simulink model "TorqueControl_QuadRad_MPC_03_FMINCON"  (R2015b)
settings: Solver=FixedStepAuto  StartTime=0.0  StopTime=100  FixedStep=1  RelTol=1e-3
values from neighbouring files (symbols this model uses):
  bicycle = initBicycle(60, 0.01468, 0.79, 0.33, 0.17, 5.5, 24, 50, 48)    [RunSimulinkSim_MPC.m]
  cyclist = initCyclist(0, 30, 183, 75, 80)    [RunSimulinkSim_MPC.m]
  environment = initEnvironment_V2(altitude, distance, fRES, 9.81, 1.2041)    [RunSimulinkSim_MPC.m]
  system = initHRmodel(0.0113, 0.0072, 0.0049, 0.0041, 19.8002, 0.0072, cyclist.P_max, cyclist.cadence)    [RunSimulinkSim_MPC.m]
undefined symbols (not defined in the file or in its folder): init
libraries: simulink x2, aerolibconvert2 x1
settings Model: Creator=Daniel  LastModifiedBy=Daniel
settings DataIOCC: SaveFormat=Array

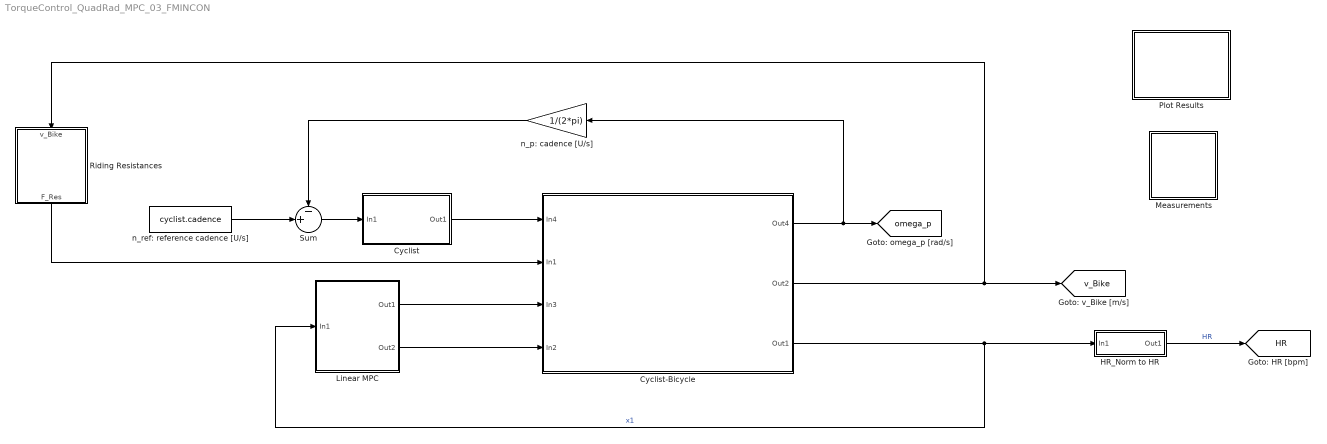
== system TorqueControl_QuadRad_MPC_03_FMINCON ==
  Cyclist : Subsystem
  Cyclist-Bicycle : Subsystem
  HR_Norm to HR : Subsystem
  Linear MPC : Subsystem
  Measurements : Subsystem
  Plot Results : Subsystem
  Riding Resistances : Subsystem
  Sum : Sum  Inputs=-+|
  n_p: cadence [U/s] : Gain  Gain=1/(2*pi)
  n_ref: reference cadence [U/s] : Constant  Value=cyclist.cadence
  tag scope: HR=global, omega_p=global, v_Bike=global
  wires:
  Linear MPC/1(Out1) -> Cyclist-Bicycle/3(In3)
  Cyclist-Bicycle/1(Out4) -> n_p: cadence [U/s]/1, [omega_p]
  n_ref: reference cadence [U/s]/1 -> Sum/2
  n_p: cadence [U/s]/1 -> Sum/1
  Riding Resistances/1(F_Res) -> Cyclist-Bicycle/2(In1)
  Cyclist-Bicycle/2(Out2) -> [v_Bike], Riding Resistances/1(v_Bike)
  Cyclist-Bicycle/3(Out1) -> Linear MPC/1(In1), HR_Norm to HR/1(In1)  "x1"
  HR_Norm to HR/1(Out1) -> [HR]  "HR"
  Sum/1 -> Cyclist/1(In1)
  Cyclist/1(Out1) -> Cyclist-Bicycle/1(In4)
  Linear MPC/2(Out2) -> Cyclist-Bicycle/4(In2)

== system TorqueControl_QuadRad_MPC_03_FMINCON/Cyclist ==
  In1 : Inport
  T_R,p: Rider torque at pedals [Nm] : simulink/Continuous/PID Controller  Controller=PID  TimeDomain=Continuous-time  SampleTime=-1  IntegratorMethod=Forward Euler  FilterMethod=Forward Euler  Form=Parallel  UseFilter=on  ControllerParametersSource=internal  P=200  I=2  D=0  N=1  InitialConditionSource=internal  InitialConditionForIntegrator=0  InitialConditionForFilter=0  ExternalReset=none  LimitOutput=on  UpperSaturationLimit=cyclist.P_max/(2*pi*2/3)  LowerSaturationLimit=0  LinearizeAsGain=on  AntiWindupMode=none  Kb=1  TrackingMode=off  Kt=1  PParamMin=[]  PParamMax=[]  IParamMin=[]  IParamMax=[]  DParamMin=[]  DParamMax=[]  NParamMin=[]  NParamMax=[]  KbParamMin=[]  KbParamMax=[]  KtParamMin=[]  KtParamMax=[]  POutMin=[]  POutMax=[]  IOutMin=[]  IOutMax=[]  DOutMin=[]  DOutMax=[]  NOutMin=[]  NOutMax=[]  KbOutMin=[]  KbOutMax=[]  KtOutMin=[]  KtOutMax=[]  IntegratorOutMin=[]  IntegratorOutMax=[]  FilterOutMin=[]  FilterOutMax=[]  SumOutMin=[]  SumOutMax=[]  SumI1OutMin=[]  SumI1OutMax=[]  SumI2OutMin=[]  SumI2OutMax=[]  SumI3OutMin=[]  SumI3OutMax=[]  SumDOutMin=[]  SumDOutMax=[]  SaturationOutMin=[]  SaturationOutMax=[]  IntegratorContinuousStateAttributes=''  IntegratorStateMustResolveToSignalObject=off  IntegratorRTWStateStorageClass=Auto  FilterContinuousStateAttributes=''  FilterStateMustResolveToSignalObject=off  FilterRTWStateStorageClass=Auto  DifferentiatorICPrevScaledInput=0  DifferentiatorOutMin=[]  DifferentiatorOutMax=[]
  Out1 : Outport
  tag scope: T_Rp=global
  wires:
  In1/1 -> T_R,p: Rider torque at pedals [Nm]/1  "e_n"
  T_R,p: Rider torque at pedals [Nm]/1 -> [T_Rp], Out1/1  "T_R,p [Nm]"

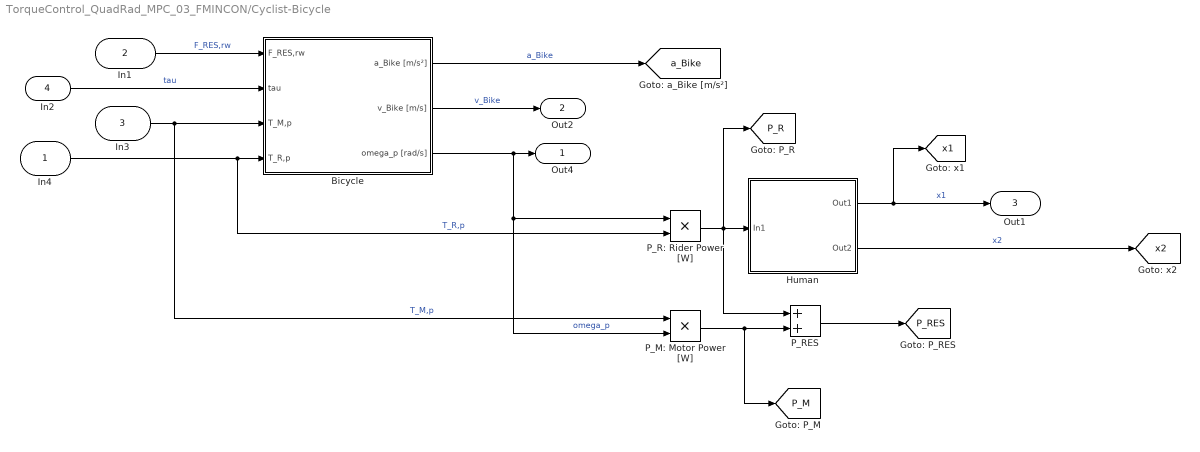
== system TorqueControl_QuadRad_MPC_03_FMINCON/Cyclist-Bicycle ==
  In4 : Inport
  In1 : Inport  Port=2
  In3 : Inport  Port=3
  In2 : Inport  Port=4
  Bicycle : Subsystem
  Human : Subsystem
  P_M: Motor Power [W] : Product
  P_R: Rider Power [W] : Product
  P_RES : Sum
  Out4 : Outport
  Out2 : Outport  Port=2
  Out1 : Outport  Port=3
  tag scope: P_M=global, P_R=global, P_RES=global, a_Bike=global, x1=global, x2=global
  wires:
  P_R: Rider Power [W]/1 -> [P_R], P_RES/1, Human/1(In1)
  Bicycle/2(v_Bike [m/s]) -> Out2/1  "v_Bike"
  Bicycle/1(a_Bike [m/s²]) -> [a_Bike]  "a_Bike"
  Human/2(Out2) -> [x2]  "x2"
  In2/1 -> Bicycle/2(tau)  "tau"
  In3/1 -> P_M: Motor Power [W]/1, Bicycle/3(T_M,p)  "T_M,p"
  In4/1 -> P_R: Rider Power [W]/2, Bicycle/4(T_R,p)  "T_R,p"
  In1/1 -> Bicycle/1(F_RES,rw)  "F_RES,rw"
  Bicycle/3(omega_p [rad/s]) -> Out4/1, P_M: Motor Power [W]/2, P_R: Rider Power [W]/1  "omega_p"
  Human/1(Out1) -> Out1/1, [x1]  "x1"
  P_M: Motor Power [W]/1 -> [P_M], P_RES/2
  P_RES/1 -> [P_RES]

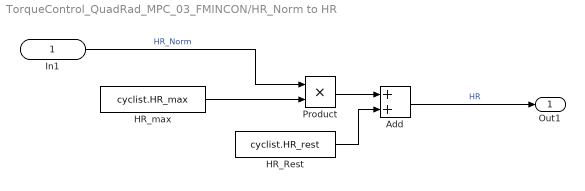
== system TorqueControl_QuadRad_MPC_03_FMINCON/HR_Norm to HR ==
  In1 : Inport
  Add : Sum
  HR_Rest : Constant  Value=cyclist.HR_rest
  HR_max : Constant  Value=cyclist.HR_max
  Product : Product
  Out1 : Outport
  wires:
  HR_max/1 -> Product/2
  Add/1 -> Out1/1  "HR"
  Product/1 -> Add/1
  HR_Rest/1 -> Add/2
  In1/1 -> Product/1  "HR_Norm"

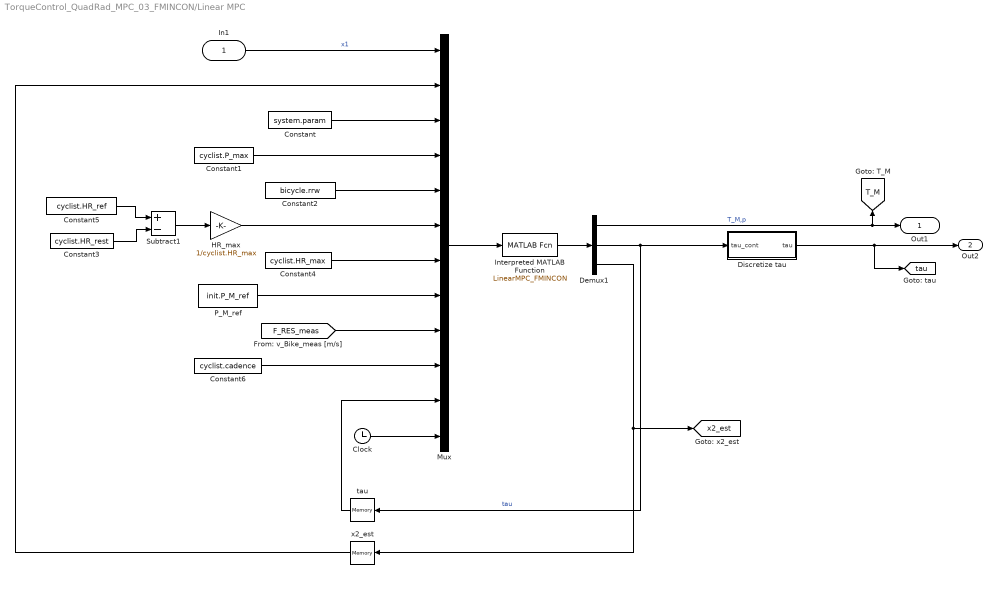
== system TorqueControl_QuadRad_MPC_03_FMINCON/Linear MPC ==
  In1 : Inport
  Clock : Clock
  Constant : Constant  Value=system.param
  Constant1 : Constant  Value=cyclist.P_max
  Constant2 : Constant  Value=bicycle.rrw
  Constant3 : Constant  Value=cyclist.HR_rest
  Constant4 : Constant  Value=cyclist.HR_max
  Constant5 : Constant  Value=cyclist.HR_ref
  Constant6 : Constant  Value=cyclist.cadence
  Demux1 : Demux  Outputs=3
  Discretize tau : MATLAB Function  TreatAsAtomicUnit=on
  HR_max : Gain  Gain=1/cyclist.HR_max
  Interpreted MATLAB Function : MATLABFcn  MATLABFcn=LinearMPC_FMINCON  OutputDimensions=3
  Mux : Mux  Inputs=12
  P_M_ref : Constant  Value=init.P_M_ref
  Subtract1 : Sum  Inputs=+-
  tau : Memory  X0=init.tau  InheritSampleTime=on
  x2_est : Memory  X0=init.x2_est  InheritSampleTime=on
  Out1 : Outport
  Out2 : Outport  Port=2
  tag scope: T_M=global, tau=global, x2_est=global
  wires:
  In1/1 -> Mux/1  "x1"
  Constant/1 -> Mux/3
  Constant1/1 -> Mux/4
  Constant2/1 -> Mux/5
  Constant5/1 -> Subtract1/1
  Constant3/1 -> Subtract1/2
  Mux/1 -> Interpreted MATLAB Function/1
  Interpreted MATLAB Function/1 -> Demux1/1
  Demux1/3 -> x2_est/1, [x2_est]
  x2_est/1 -> Mux/2
  P_M_ref/1 -> Mux/8
  [F_RES_meas] -> Mux/9
  Constant6/1 -> Mux/10
  Subtract1/1 -> HR_max/1
  HR_max/1 -> Mux/6
  Demux1/1 -> Out1/1, [T_M]  "T_M,p"
  Demux1/2 -> tau/1, Discretize tau/1(tau_cont)  "tau"
  tau/1 -> Mux/11
  Constant4/1 -> Mux/7
  Clock/1 -> Mux/12
  Discretize tau/1(tau) -> Out2/1, [tau]

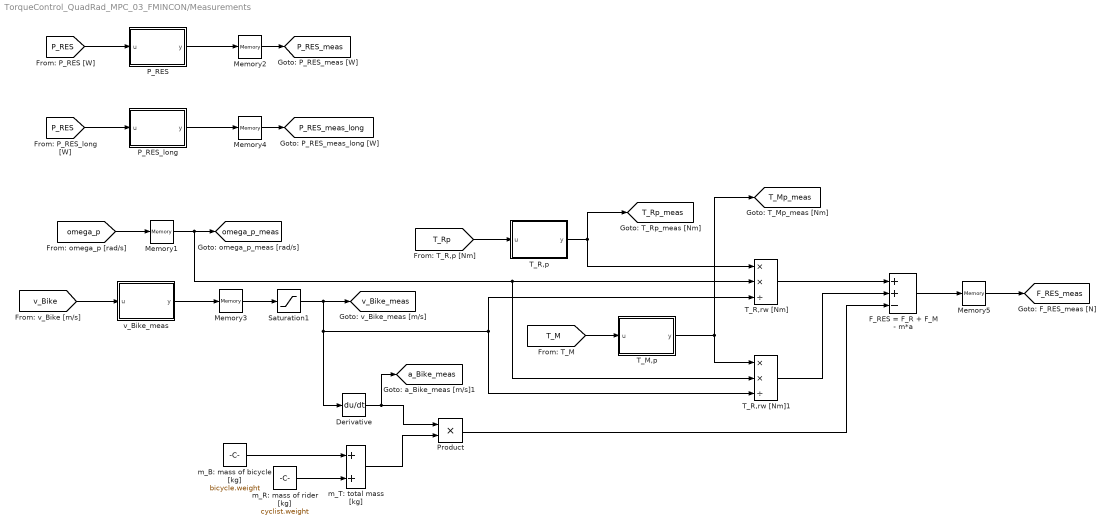
== system TorqueControl_QuadRad_MPC_03_FMINCON/Measurements ==
  Derivative : Derivative
  F_RES = F_R + F_M - m*a : Sum  Inputs=++-
  Memory1 : Memory  X0=init.omega_p  InheritSampleTime=on
  Memory2 : Memory  X0=init.P_RES  InheritSampleTime=on
  Memory3 : Memory  X0=init.v_Bike  InheritSampleTime=on
  Memory4 : Memory  X0=init.P_RES  InheritSampleTime=on
  Memory5 : Memory  X0=10  InheritSampleTime=on
  P_RES : MATLAB Function  TreatAsAtomicUnit=on
  P_RES_long : MATLAB Function  TreatAsAtomicUnit=on
  Product : Product
  Saturation1 : Saturate  UpperLimit=100  LowerLimit=0.1
  T_M,p : MATLAB Function  TreatAsAtomicUnit=on
  T_R,p : MATLAB Function  TreatAsAtomicUnit=on
  T_R,rw [Nm] : Product  Inputs=**/
  T_R,rw [Nm]1 : Product  Inputs=**/
  m_B: mass of bicycle [kg] : Constant  Value=bicycle.weight
  m_R: mass of rider [kg] : Constant  Value=cyclist.weight
  m_T: total mass [kg] : Sum
  v_Bike_meas : MATLAB Function  TreatAsAtomicUnit=on
  tag scope: F_RES_meas=global, P_RES_meas=global, P_RES_meas_long=global, T_Mp_meas=global, T_Rp_meas=global, a_Bike_meas=global, omega_p_meas=global, v_Bike_meas=global
  wires:
  [P_RES] -> P_RES/1(u)
  Memory2/1 -> [P_RES_meas]
  [omega_p] -> Memory1/1
  Memory1/1 -> T_R,rw [Nm]1/2, T_R,rw [Nm]/2, [omega_p_meas]
  P_RES/1(y) -> Memory2/1
  Memory3/1 -> Saturation1/1
  [v_Bike] -> v_Bike_meas/1(u)
  Saturation1/1 -> T_R,rw [Nm]1/3, T_R,rw [Nm]/3, Derivative/1, [v_Bike_meas]
  v_Bike_meas/1(y) -> Memory3/1
  [P_RES] -> P_RES_long/1(u)
  Memory4/1 -> [P_RES_meas_long]
  P_RES_long/1(y) -> Memory4/1
  m_B: mass of bicycle [kg]/1 -> m_T: total mass [kg]/1
  m_T: total mass [kg]/1 -> Product/2
  m_R: mass of rider [kg]/1 -> m_T: total mass [kg]/2
  Derivative/1 -> [a_Bike_meas], Product/1
  [T_Rp] -> T_R,p/1(u)
  [T_M] -> T_M,p/1(u)
  T_R,rw [Nm]/1 -> F_RES = F_R + F_M - m*a/1
  T_R,rw [Nm]1/1 -> F_RES = F_R + F_M - m*a/2
  Product/1 -> F_RES = F_R + F_M - m*a/3
  F_RES = F_R + F_M - m*a/1 -> Memory5/1
  Memory5/1 -> [F_RES_meas]
  T_R,p/1(y) -> T_R,rw [Nm]/1, [T_Rp_meas]
  T_M,p/1(y) -> T_R,rw [Nm]1/1, [T_Mp_meas]

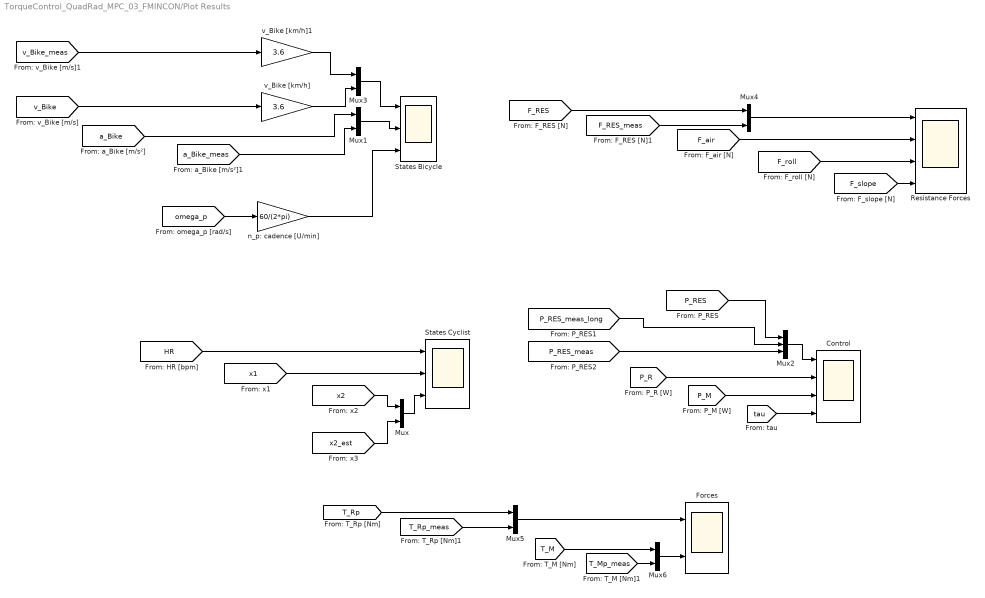
== system TorqueControl_QuadRad_MPC_03_FMINCON/Plot Results ==
  Control : Scope  NumInputPorts=4
  Forces : Scope  NumInputPorts=2
  Mux{,1,3..6} (6 alike) : Mux  Inputs=2
  Mux2 : Mux  Inputs=3
  Resistance Forces : Scope  NumInputPorts=4
  States Bicycle : Scope  NumInputPorts=3
  States Cyclist : Scope  NumInputPorts=3
  n_p: cadence [U/min] : Gain  Gain=60/(2*pi)
  v_Bike [km/h] : Gain  Gain=3.6
  v_Bike [km/h]1 : Gain  Gain=3.6
  wires:
  [omega_p] -> n_p: cadence [U/min]/1
  [v_Bike] -> v_Bike [km/h]/1
  n_p: cadence [U/min]/1 -> States Bicycle/3
  [HR] -> States Cyclist/1
  [x1] -> States Cyclist/2
  [x2] -> Mux/1
  v_Bike [km/h]/1 -> Mux3/2
  [F_RES] -> Mux4/1
  [F_air] -> Resistance Forces/2
  [F_roll] -> Resistance Forces/3
  [F_slope] -> Resistance Forces/4
  [T_M] -> Mux6/1
  [P_M] -> Control/3
  [P_RES] -> Mux2/1
  [T_Rp] -> Mux5/1
  [x2_est] -> Mux/2
  Mux/1 -> States Cyclist/3
  [tau] -> Control/4
  Mux2/1 -> Control/1
  [P_RES_meas_long] -> Mux2/2
  [P_RES_meas] -> Mux2/3
  [v_Bike_meas] -> v_Bike [km/h]1/1
  v_Bike [km/h]1/1 -> Mux3/1
  Mux3/1 -> States Bicycle/1
  [F_RES_meas] -> Mux4/2
  Mux4/1 -> Resistance Forces/1
  [a_Bike] -> Mux1/1
  [a_Bike_meas] -> Mux1/2
  Mux1/1 -> States Bicycle/2
  [T_Rp_meas] -> Mux5/2
  Mux5/1 -> Forces/1
  Mux6/1 -> Forces/2
  [T_Mp_meas] -> Mux6/2
  [P_R] -> Control/2

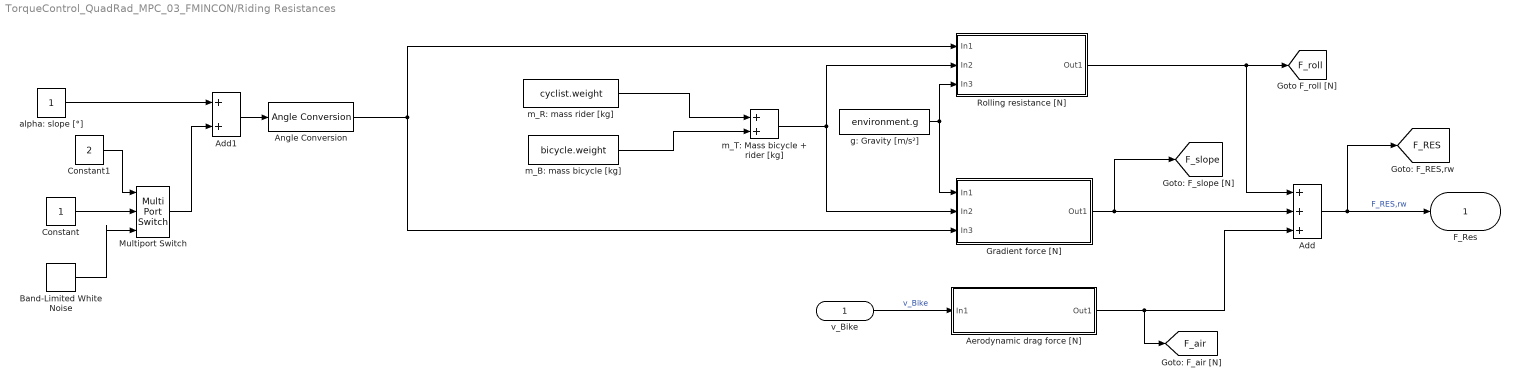
== system TorqueControl_QuadRad_MPC_03_FMINCON/Riding Resistances ==
  v_Bike : Inport
  Add : Sum  Inputs=+++
  Add1 : Sum
  Aerodynamic drag force [N] : Subsystem
  Angle Conversion : aerolibconvert2/Angle Conversion  IU=deg  OU=rad
  Band-Limited White Noise : simulink/Sources/Band-Limited White Noise  Cov=[0.1]  Ts=1  seed=[23341]
  Constant : Constant
  Constant1 : Constant  Value=2
  Gradient force [N] : Subsystem
  Multiport Switch : MultiPortSwitch  Inputs=2
  Rolling resistance [N] : Subsystem
  alpha: slope [°] : Constant
  g: Gravity [m/s²] : Constant  Value=environment.g
  m_B: mass bicycle [kg] : Constant  Value=bicycle.weight
  m_R: mass rider [kg] : Constant  Value=cyclist.weight
  m_T: Mass bicycle + rider [kg] : Sum
  F_Res : Outport
  tag scope: F_RES=global, F_air=global, F_roll=global, F_slope=global
  wires:
  Gradient force [N]/1(Out1) -> [F_slope], Add/2
  Aerodynamic drag force [N]/1(Out1) -> [F_air], Add/3
  v_Bike/1 -> Aerodynamic drag force [N]/1(In1)  "v_Bike"
  Angle Conversion/1 -> Gradient force [N]/3(In3), Rolling resistance [N]/1(In1)
  Add/1 -> [F_RES], F_Res/1  "F_RES,rw"
  g: Gravity [m/s²]/1 -> Rolling resistance [N]/3(In3), Gradient force [N]/1(In1)
  m_T: Mass bicycle + rider [kg]/1 -> Gradient force [N]/2(In2), Rolling resistance [N]/2(In2)
  m_R: mass rider [kg]/1 -> m_T: Mass bicycle + rider [kg]/1
  m_B: mass bicycle [kg]/1 -> m_T: Mass bicycle + rider [kg]/2
  alpha: slope [°]/1 -> Add1/1
  Rolling resistance [N]/1(Out1) -> Add/1, [F_roll]
  Band-Limited White Noise/1 -> Multiport Switch/3
  Add1/1 -> Angle Conversion/1
  Constant/1 -> Multiport Switch/2
  Constant1/1 -> Multiport Switch/1
  Multiport Switch/1 -> Add1/2

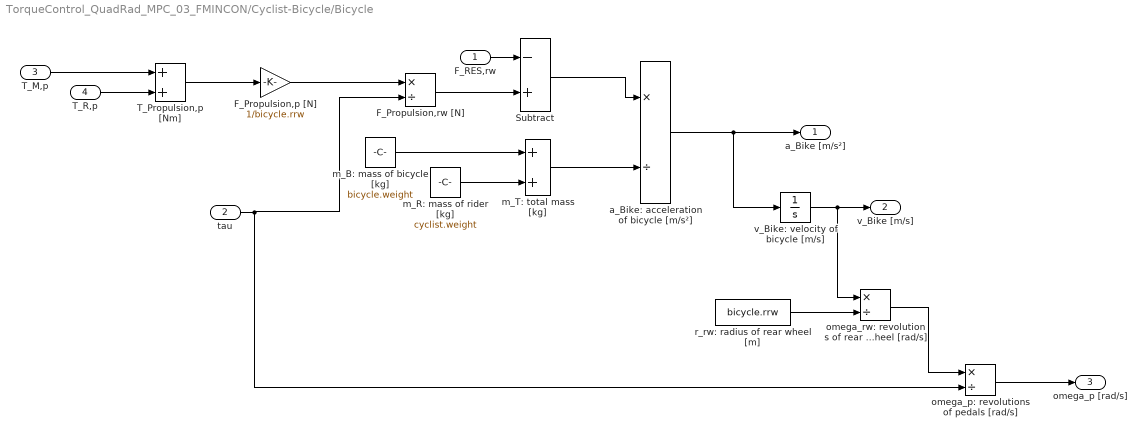
== system TorqueControl_QuadRad_MPC_03_FMINCON/Cyclist-Bicycle/Bicycle ==
  F_RES,rw : Inport
  tau : Inport  Port=2
  T_M,p : Inport  Port=3
  T_R,p : Inport  Port=4
  F_Propulsion,p [N] : Gain  Gain=1/bicycle.rrw
  F_Propulsion,rw [N] : Product  Inputs=*/
  Subtract : Sum  Inputs=-+
  T_Propulsion,p [Nm] : Sum
  a_Bike: acceleration of bicycle [m/s²] : Product  Inputs=*/
  m_B: mass of bicycle [kg] : Constant  Value=bicycle.weight
  m_R: mass of rider [kg] : Constant  Value=cyclist.weight
  m_T: total mass [kg] : Sum
  omega_p: revolutions of pedals [rad/s] : Product  Inputs=*/
  omega_rw: revolutions of rear wheel [rad/s] : Product  Inputs=*/
  r_rw: radius of rear wheel [m] : Constant  Value=bicycle.rrw
  v_Bike: velocity of bicycle [m/s] : Integrator  InitialCondition=init.v_Bike
  a_Bike [m/s²] : Outport
  v_Bike [m/s] : Outport  Port=2
  omega_p [rad/s] : Outport  Port=3
  wires:
  m_B: mass of bicycle [kg]/1 -> m_T: total mass [kg]/1
  T_R,p/1 -> T_Propulsion,p [Nm]/2
  a_Bike: acceleration of bicycle [m/s²]/1 -> a_Bike [m/s²]/1, v_Bike: velocity of bicycle [m/s]/1
  m_T: total mass [kg]/1 -> a_Bike: acceleration of bicycle [m/s²]/2
  m_R: mass of rider [kg]/1 -> m_T: total mass [kg]/2
  T_M,p/1 -> T_Propulsion,p [Nm]/1
  F_RES,rw/1 -> Subtract/1
  tau/1 -> F_Propulsion,rw [N]/2, omega_p: revolutions of pedals [rad/s]/2
  Subtract/1 -> a_Bike: acceleration of bicycle [m/s²]/1
  r_rw: radius of rear wheel [m]/1 -> omega_rw: revolutions of rear wheel [rad/s]/2
  v_Bike: velocity of bicycle [m/s]/1 -> omega_rw: revolutions of rear wheel [rad/s]/1, v_Bike [m/s]/1
  omega_rw: revolutions of rear wheel [rad/s]/1 -> omega_p: revolutions of pedals [rad/s]/1
  omega_p: revolutions of pedals [rad/s]/1 -> omega_p [rad/s]/1
  T_Propulsion,p [Nm]/1 -> F_Propulsion,p [N]/1
  F_Propulsion,p [N]/1 -> F_Propulsion,rw [N]/1
  F_Propulsion,rw [N]/1 -> Subtract/2

== system TorqueControl_QuadRad_MPC_03_FMINCON/Cyclist-Bicycle/Human ==
  In1 : Inport
  Nonlinear Human Model : Subsystem
  Power to Power_Norm : Subsystem
  Out1 : Outport
  Out2 : Outport  Port=2
  wires:
  In1/1 -> Power to Power_Norm/1(In1)  "P_Rider"
  Nonlinear Human Model/1(Out1) -> Out1/1  "x1"
  Nonlinear Human Model/2(Out2) -> Out2/1  "x2"
  Power to Power_Norm/1(Out1) -> Nonlinear Human Model/1(In1)

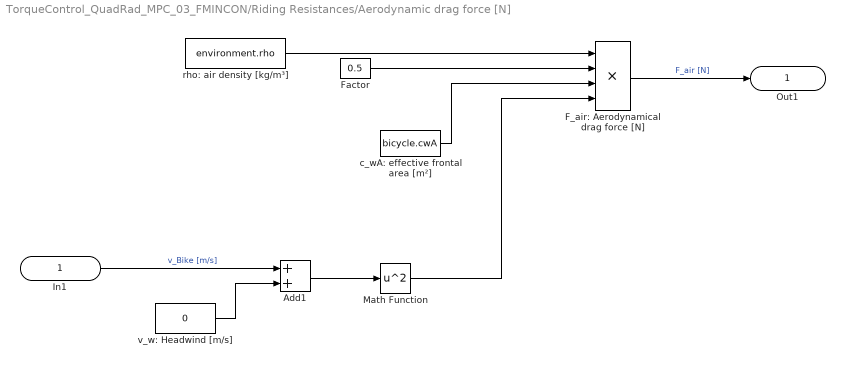
== system TorqueControl_QuadRad_MPC_03_FMINCON/Riding Resistances/Aerodynamic drag force [N] ==
  In1 : Inport
  Add1 : Sum
  F_air: Aerodynamical drag force [N] : Product  Inputs=4
  Factor : Constant  Value=0.5
  Math Function : Math  Operator=square  SaturateOnIntegerOverflow=on
  "c_wA: effective frontal area [m²] " : Constant  Value=bicycle.cwA
  rho: air density [kg/m³] : Constant  Value=environment.rho
  v_w: Headwind [m/s] : Constant  Value=0
  Out1 : Outport
  wires:
  v_w: Headwind [m/s]/1 -> Add1/2
  Add1/1 -> Math Function/1
  "c_wA: effective frontal area [m²] "/1 -> F_air: Aerodynamical drag force [N]/3
  In1/1 -> Add1/1  "v_Bike [m/s]"
  Factor/1 -> F_air: Aerodynamical drag force [N]/2
  rho: air density [kg/m³]/1 -> F_air: Aerodynamical drag force [N]/1
  F_air: Aerodynamical drag force [N]/1 -> Out1/1  "F_air [N]"
  Math Function/1 -> F_air: Aerodynamical drag force [N]/4

== system TorqueControl_QuadRad_MPC_03_FMINCON/Riding Resistances/Gradient force [N] ==
  In1 : Inport
  In2 : Inport  Port=2
  In3 : Inport  Port=3
  F_slope: Gradient force [N] : Product  Inputs=3
  Trigonometric Function : Trigonometry
  Out1 : Outport
  wires:
  In1/1 -> F_slope: Gradient force [N]/1  "g [m/s²]"
  In3/1 -> Trigonometric Function/1  "alpha [rad]"
  In2/1 -> F_slope: Gradient force [N]/2  "m_T [kg]"
  Trigonometric Function/1 -> F_slope: Gradient force [N]/3
  F_slope: Gradient force [N]/1 -> Out1/1  "F_slope [N]"

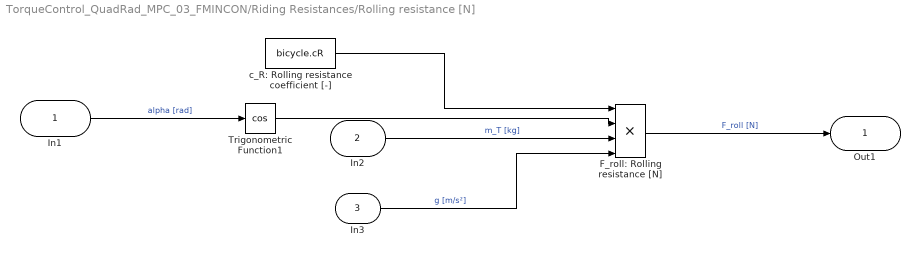
== system TorqueControl_QuadRad_MPC_03_FMINCON/Riding Resistances/Rolling resistance [N] ==
  In1 : Inport
  In2 : Inport  Port=2
  In3 : Inport  Port=3
  F_roll: Rolling resistance [N] : Product  Inputs=4
  Trigonometric Function1 : Trigonometry  Operator=cos
  c_R: Rolling resistance coefficient [-] : Constant  Value=bicycle.cR
  Out1 : Outport
  wires:
  In1/1 -> Trigonometric Function1/1  "alpha [rad]"
  In3/1 -> F_roll: Rolling resistance [N]/4  "g [m/s²]"
  In2/1 -> F_roll: Rolling resistance [N]/3  "m_T [kg]"
  c_R: Rolling resistance coefficient [-]/1 -> F_roll: Rolling resistance [N]/1
  Trigonometric Function1/1 -> F_roll: Rolling resistance [N]/2
  F_roll: Rolling resistance [N]/1 -> Out1/1  "F_roll [N]"

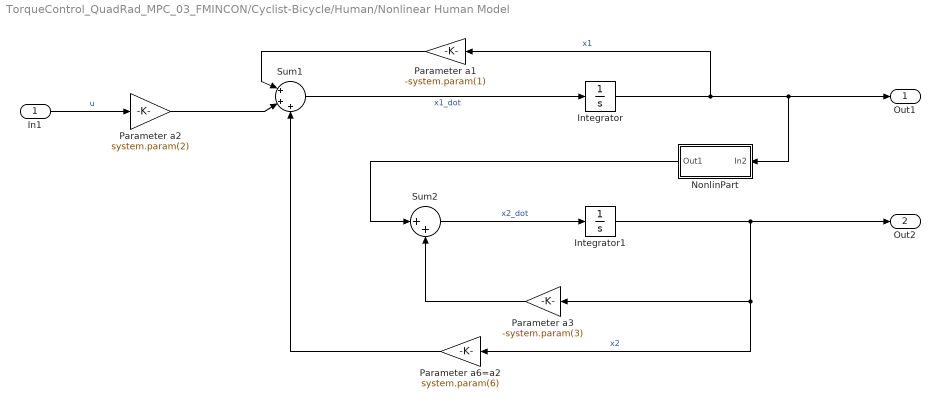
== system TorqueControl_QuadRad_MPC_03_FMINCON/Cyclist-Bicycle/Human/Nonlinear Human Model ==
  In1 : Inport
  Integrator : Integrator  InitialCondition=init.x1
  Integrator1 : Integrator  InitialCondition=init.x2
  NonlinPart : Subsystem
  Parameter a1 : Gain  Gain=-system.param(1)
  Parameter a2 : Gain  Gain=system.param(2)
  Parameter a3 : Gain  Gain=-system.param(3)
  Parameter a6=a2 : Gain  Gain=system.param(6)
  Sum1 : Sum  Inputs=|+++
  Sum2 : Sum  Inputs=|++
  Out1 : Outport
  Out2 : Outport  Port=2
  wires:
  Integrator/1 -> Parameter a1/1, Out1/1, NonlinPart/1(In2)  "x1"
  Integrator1/1 -> Parameter a6=a2/1, Parameter a3/1, Out2/1  "x2"
  Parameter a6=a2/1 -> Sum1/3
  NonlinPart/1(Out1) -> Sum2/1
  Sum2/1 -> Integrator1/1  "x2_dot"
  Parameter a3/1 -> Sum2/2
  Parameter a1/1 -> Sum1/1
  In1/1 -> Parameter a2/1  "u"
  Sum1/1 -> Integrator/1  "x1_dot"
  Parameter a2/1 -> Sum1/2

== system TorqueControl_QuadRad_MPC_03_FMINCON/Cyclist-Bicycle/Human/Power to Power_Norm ==
  In1 : Inport
  Constant : Constant  Value=cyclist.P_max
  Divide : Product  Inputs=*/
  Saturation : Saturate  UpperLimit=cyclist.P_max  LowerLimit=0  ZeroCross=off
  Out1 : Outport
  wires:
  Constant/1 -> Divide/2
  Divide/1 -> Out1/1  "Power_Norm"
  In1/1 -> Saturation/1  "Power"
  Saturation/1 -> Divide/1

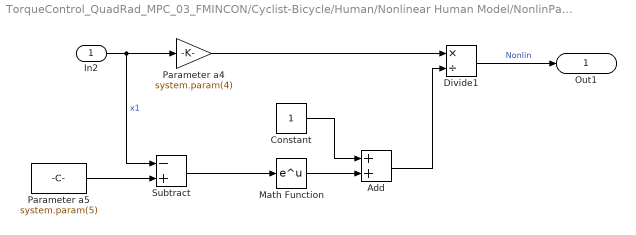
== system TorqueControl_QuadRad_MPC_03_FMINCON/Cyclist-Bicycle/Human/Nonlinear Human Model/NonlinPart ==
  In2 : Inport
  Add : Sum
  Constant : Constant
  Divide1 : Product  Inputs=*/
  Math Function : Math  SaturateOnIntegerOverflow=on
  Parameter a4 : Gain  Gain=system.param(4)
  Parameter a5 : Constant  Value=system.param(5)
  Subtract : Sum  Inputs=-+
  Out1 : Outport
  wires:
  Parameter a4/1 -> Divide1/1
  In2/1 -> Subtract/1, Parameter a4/1  "x1"
  Divide1/1 -> Out1/1  "Nonlin"
  Constant/1 -> Add/1
  Parameter a5/1 -> Subtract/2
  Math Function/1 -> Add/2
  Add/1 -> Divide1/2
  Subtract/1 -> Math Function/1

== matlab function TorqueControl_QuadRad_MPC_03_FMINCON/Linear MPC/Discretize tau ==
  data: tau_cont input; tau output
function tau = fcn(tau_cont)
%#codegen

if tau_cont>2.3
    tau = 2.5;
elseif tau_cont>2.0
    tau = 2.1;
elseif tau_cont>1.8
    tau = 1.9;
elseif tau_cont>1.6
    tau = 1.7;
elseif tau_cont>1.4
    tau = 1.5;
elseif tau_cont>1.2
    tau = 1.3;
else
    tau = 1.1;
end

== matlab function TorqueControl_QuadRad_MPC_03_FMINCON/Measurements/P_RES ==
  data: u input; y output
function y = fcn(u)
%#codegen
persistent i buf bufSum;
if isempty(buf)
    buf = zeros(1,5);
    bufSum = 0;
    i = 1;
end
bufSum = bufSum - buf(i);
buf(i) = u;
bufSum = bufSum + u;
i = i + 1;
if i > numel(buf)
    i = 1;
end
y = bufSum / numel(buf);

== matlab function TorqueControl_QuadRad_MPC_03_FMINCON/Measurements/v_Bike_meas ==
  data: u input; y output
function y = fcn(u)
%#codegen
persistent i3 buf3 bufSum3;
if isempty(buf3)
    buf3 = zeros(1,5);
    bufSum3 = 0;
    i3 = 1;
end
bufSum3 = bufSum3 - buf3(i3);
buf3(i3) = u;
bufSum3 = bufSum3 + u;
i3 = i3 + 1;
if i3 > numel(buf3)
    i3 = 1;
end
y = bufSum3 / numel(buf3);

== matlab function TorqueControl_QuadRad_MPC_03_FMINCON/Measurements/P_RES_long ==
  data: u input; y output
function y = fcn(u)
%#codegen
persistent i2 buf2 bufSum2;
if isempty(buf2)
    buf2 = zeros(1,60);
    bufSum2 = 0;
    i2 = 1;
end
bufSum2 = bufSum2 - buf2(i2);
buf2(i2) = u;
bufSum2 = bufSum2 + u;
i2 = i2 + 1;
if i2 > numel(buf2)
    i2 = 1;
end
num = numel(buf2);
y = bufSum2/num;

== matlab function TorqueControl_QuadRad_MPC_03_FMINCON/Measurements/T_R,p ==
  data: u input; y output
function y = fcn(u)
%#codegen
persistent i buf bufSum;
if isempty(buf)
    buf = zeros(1,10);
    bufSum = 0;
    i = 1;
end
bufSum = bufSum - buf(i);
buf(i) = u;
bufSum = bufSum + u;
i = i + 1;
if i > numel(buf)
    i = 1;
end
y = bufSum / numel(buf);

== matlab function TorqueControl_QuadRad_MPC_03_FMINCON/Measurements/T_M,p ==
  data: u input; y output
function y = fcn(u)
%#codegen
persistent i buf bufSum;
if isempty(buf)
    buf = zeros(1,5);
    bufSum = 0;
    i = 1;
end
bufSum = bufSum - buf(i);
buf(i) = u;
bufSum = bufSum + u;
i = i + 1;
if i > numel(buf)
    i = 1;
end
y = bufSum / numel(buf);
